simulink model "valo_FR"  (R2022a)
settings: Solver=VariableStepAuto  StartTime=0.0  StopTime=10.0  RelTol=1e-3
libraries: Assets x3, simulink x1
settings Model: Creator=a.dehghan  LastModifiedBy=a.dehghan

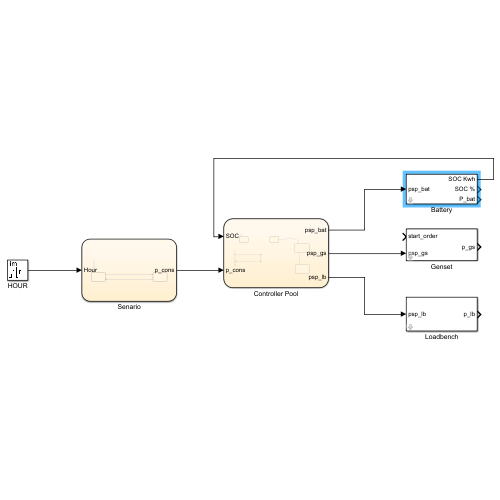
[thumbnail: Simulink's stored preview of the top-level diagram]
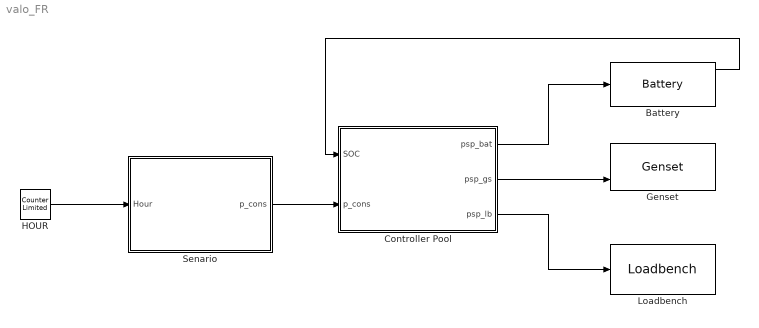
== system valo_FR ==
  Battery : Assets/Battery  max_soc_limit=max_soc_limit  min_soc_limit=min_soc_limit  efficiency_discharge=efficiency_discharge  efficiency_charge=efficiency_charge  psp_bat=p
      settings: SourceProductName=My Library
  Controller Pool : Stateflow chart  TreatAsAtomicUnit=on
  Genset : Assets/Genset  start_order=[0 1]  psp_PE=psp_EP  t=t
      settings: SourceProductName=My Library
  HOUR : simulink/Sources/Counter Limited  uplimit=24  tsamp=1
  Loadbench : Assets/Loadbench  psp_lb=psp_lb
      settings: SourceProductName=My Library
  Senario : Stateflow chart  TreatAsAtomicUnit=on
  wires:
  HOUR/1 -> Senario/1(Hour)
  Controller Pool/1(psp_bat) -> Battery/1
  Controller Pool/2(psp_gs) -> Genset/2
  Controller Pool/3(psp_lb) -> Loadbench/1
  Senario/1(p_cons) -> Controller Pool/2(p_cons)
  Battery/1 -> Controller Pool/1(SOC)

== stateflow chart valo_FR/Controller Pool ==
  state ?
  state Genset
    entry : p_cons = psp_gs;
    during : psp_lb = 0;
    exit :
  state Battery
    entry : p_cons = psp_bat;
    during : psp_gs = 0 , psp_lb = 0;
    exit : min_soc > SOC < max_soc;
  state Genset1
    entry:
    counter = 0;
    during:
    counter = counter + 1;
  state ? [function]
    (default) -> (junction 51)
  state Loadbench
    entry : psp_gs = 0;
    psp_lb = psp_lb;
  (default) -> (junction 56) [order 2]
  (default) -> Battery [order 1] : [min_soc < SOC > max_soc]
  (junction 56) -> ? [order 2] : [SOC > max_soc]
  Genset -> Battery : [SOC > min_soc]
  (junction 56) -> Genset1 [order 1] : [SOC < min_soc && counter > 10]
  Battery -> Genset [order 1] : [SOC < min_soc && psp >=0]
  Battery -> Loadbench [order 2] : [SOC > max_soc && psp <=0]
  Loadbench -> Battery : [SOC < max_soc]
  (junction 41) -> (junction 42) [order 1] : [soc < min_soc ,  psp >=0]
  (junction 41) -> (junction 43) [order 2] : {psps_gs = 0 , psp_lb = 0, hysteresis = 0;}
  (junction 42) -> (junction 44) : {psps_gs = psp_gs , psp_lb = 0, hysteresis = -1;}
  (junction 44) -> (junction 43)
  (junction 43) -> (junction 45)
  data: SOC input; psp_bat output; psp_gs output; psp_lb output; p_cons input

== stateflow chart valo_FR/Senario ==
  state decharge
    entry : p = 5;
  state charge
    entry : p = -5
  (default) -> decharge
  decharge -> charge : [Hour >= 12 && Hour < 18]
  charge -> decharge : [Hour >=18]
  data: Hour input; p_cons output
